simulink library "IP_MASTER"  (Simulink 8.6)
settings: Solver=ode45  StartTime=0.0  StopTime=10.0  RelTol=1e-3
libraries: cdsEpicsOut x56, cdsFilt x38, cdsFiltCtrl x36, cdsEpicsIn x18, cdsTP x12, cdsMuxMatrix x7, cdsRampMuxMatrix x2, cdsFunctionCall x2, SIXOSEM_F_WD_AC_MASTER x2, SIXOSEM_F_STAGE_MASTER x2, ADV_IP_MASTER x2
(part 9 of 9)

== system IP_MASTER/IP_shutdown/SET ==
  Ground1 : Ground
  Ground2 : Ground
  Ground3 : Ground
  L : cdsFilt/Subsystem  Tag=cdsFilt  Description=|
      | Purpose:                                                                                                                                                                                                                                  
      | Standard CDS IIR filter module.                                                                                                                                                                                                           
      |                                                                                                                                                                                                                                           
      | Operation:                                                                                                                                                                                                                                
      | Consists of 10 second order section IIR filters, plus a ramped gain stage. In FE code, also provides pre-defined test points and excitation channel inputs. The filter coefficients are defined in the LIGO system using the 'foton' tool.
      |                                                                                                                                                                                                                                           
      | Usage:                                                                                                                                                                                                                                    
      | Name the part with the desired filter module name.
      settings: AttributesFormatString=%<Tag>
  T : cdsFilt/Subsystem  Tag=cdsFilt  Description=|
      | Purpose:                                                                                                                                                                                                                                  
      | Standard CDS IIR filter module.                                                                                                                                                                                                           
      |                                                                                                                                                                                                                                           
      | Operation:                                                                                                                                                                                                                                
      | Consists of 10 second order section IIR filters, plus a ramped gain stage. In FE code, also provides pre-defined test points and excitation channel inputs. The filter coefficients are defined in the LIGO system using the 'foton' tool.
      |                                                                                                                                                                                                                                           
      | Usage:                                                                                                                                                                                                                                    
      | Name the part with the desired filter module name.
      settings: AttributesFormatString=%<Tag>
  Y : cdsFilt/Subsystem  Tag=cdsFilt  Description=|
      | Purpose:                                                                                                                                                                                                                                  
      | Standard CDS IIR filter module.                                                                                                                                                                                                           
      |                                                                                                                                                                                                                                           
      | Operation:                                                                                                                                                                                                                                
      | Consists of 10 second order section IIR filters, plus a ramped gain stage. In FE code, also provides pre-defined test points and excitation channel inputs. The filter coefficients are defined in the LIGO system using the 'foton' tool.
      |                                                                                                                                                                                                                                           
      | Usage:                                                                                                                                                                                                                                    
      | Name the part with the desired filter module name.
      settings: AttributesFormatString=%<Tag>
  LONG_Out : Outport
  TRANS_Out : Outport  Port=2
  YAW_Out : Outport  Port=3
  wires:
  Ground3/1 -> Y/1
  Ground2/1 -> T/1
  Ground1/1 -> L/1
  L/1 -> LONG_Out/1
  T/1 -> TRANS_Out/1
  Y/1 -> YAW_Out/1

== system IP_MASTER/IP_shutdown/TEST ==
  Ground1 : Ground
  Ground2 : Ground
  Ground3 : Ground
  L : cdsFilt/Subsystem  Tag=cdsFilt  Description=|
      | Purpose:                                                                                                                                                                                                                                  
      | Standard CDS IIR filter module.                                                                                                                                                                                                           
      |                                                                                                                                                                                                                                           
      | Operation:                                                                                                                                                                                                                                
      | Consists of 10 second order section IIR filters, plus a ramped gain stage. In FE code, also provides pre-defined test points and excitation channel inputs. The filter coefficients are defined in the LIGO system using the 'foton' tool.
      |                                                                                                                                                                                                                                           
      | Usage:                                                                                                                                                                                                                                    
      | Name the part with the desired filter module name.
      settings: AttributesFormatString=%<Tag>
  T : cdsFilt/Subsystem  Tag=cdsFilt  Description=|
      | Purpose:                                                                                                                                                                                                                                  
      | Standard CDS IIR filter module.                                                                                                                                                                                                           
      |                                                                                                                                                                                                                                           
      | Operation:                                                                                                                                                                                                                                
      | Consists of 10 second order section IIR filters, plus a ramped gain stage. In FE code, also provides pre-defined test points and excitation channel inputs. The filter coefficients are defined in the LIGO system using the 'foton' tool.
      |                                                                                                                                                                                                                                           
      | Usage:                                                                                                                                                                                                                                    
      | Name the part with the desired filter module name.
      settings: AttributesFormatString=%<Tag>
  Y : cdsFilt/Subsystem  Tag=cdsFilt  Description=|
      | Purpose:                                                                                                                                                                                                                                  
      | Standard CDS IIR filter module.                                                                                                                                                                                                           
      |                                                                                                                                                                                                                                           
      | Operation:                                                                                                                                                                                                                                
      | Consists of 10 second order section IIR filters, plus a ramped gain stage. In FE code, also provides pre-defined test points and excitation channel inputs. The filter coefficients are defined in the LIGO system using the 'foton' tool.
      |                                                                                                                                                                                                                                           
      | Usage:                                                                                                                                                                                                                                    
      | Name the part with the desired filter module name.
      settings: AttributesFormatString=%<Tag>
  LONG_Out : Outport
  TRANS_Out : Outport  Port=2
  YAW_Out : Outport  Port=3
  wires:
  Ground3/1 -> Y/1
  Ground2/1 -> T/1
  Ground1/1 -> L/1
  L/1 -> LONG_Out/1
  T/1 -> TRANS_Out/1
  Y/1 -> YAW_Out/1

== system IP_MASTER/IP_shutdown/WD ==
  LVDT_H1_In : Inport
  LVDT_H2_In : Inport  Port=2
  LVDT_H3_In : Inport  Port=3
  ACC_H1_In : Inport  Port=4
  ACC_H2_In : Inport  Port=5
  ACC_H3_In : Inport  Port=6
  AC : SIXOSEM_F_WD_AC_MASTER/AC2THRESHOLD
  F0_AC_FLAG_Out : Outport
  wires:
  ACC_H3_In/1 -> AC/6
  ACC_H2_In/1 -> AC/5
  ACC_H1_In/1 -> AC/4
  LVDT_H3_In/1 -> AC/3
  LVDT_H2_In/1 -> AC/2
  LVDT_H1_In/1 -> AC/1
  AC/1 -> F0_AC_FLAG_Out/1
